simulink subsystem "median4"  (R2021b)
settings: Solver=VariableStepAuto  StartTime=0.0  StopTime=10.0  RelTol=1e-3
settings Model: Creator=dileepan  LastModifiedBy=dileepan

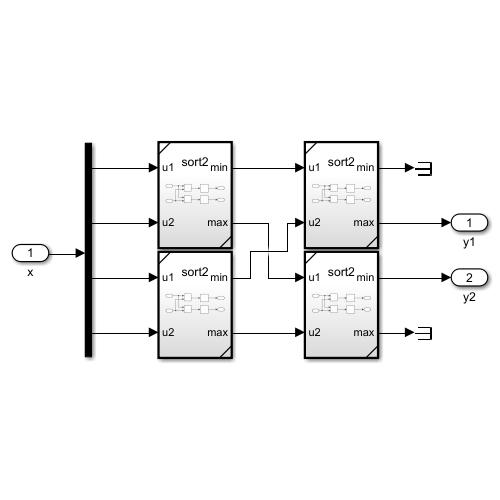
[thumbnail: Simulink's stored preview of the top-level diagram]
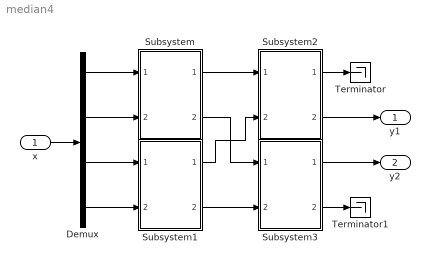
== system median4 ==
  x : Inport
  Demux : Demux
  Subsystem{,1..3} (4 alike) : Subsystem  TreatAsAtomicUnit=on  ReferencedSubsystem=sort2
  Terminator : Terminator
  Terminator1 : Terminator
  y1 : Outport
  y2 : Outport  Port=2
  wires:
  Demux/1 -> Subsystem/1
  Demux/2 -> Subsystem/2
  Subsystem/1 -> Subsystem2/1
  Subsystem1/2 -> Subsystem3/2
  Subsystem2/1 -> Terminator/1
  Subsystem3/2 -> Terminator1/1
  Subsystem2/2 -> y1/1
  Subsystem3/1 -> y2/1
  x/1 -> Demux/1
  Demux/3 -> Subsystem1/1
  Demux/4 -> Subsystem1/2
  Subsystem/2 -> Subsystem3/1
  Subsystem1/1 -> Subsystem2/2
